simulink model "Data"  (R2019b)
settings: Solver=VariableStepAuto  StartTime=0.0  StopTime=10.0  RelTol=1e-3
settings Model: Creator=Lenovo  LastModifiedBy=Lenovo
settings OptimizationCC: DefaultParameterBehavior=Inlined

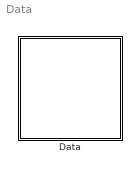
== system Data ==
  Data : Stateflow chart  BlockKeywords=__PRM__SERIALIZED__DATA__:Stateflow Chart,Stateflow Diagram  TreatAsAtomicUnit=on

== stateflow chart Data/Data ==
  state ON
  state OFF
  state StandBy
  (default) -> ON
  StandBy -> ON
  OFF -> ON [order 1]
  ON -> OFF
  OFF -> StandBy [order 2]
